simulink model "project_6"  (R2019a)
settings: Solver=VariableStepAuto  StartTime=0.0  StopTime=10.0  RelTol=1e-3
values from neighbouring files (symbols this model uses):
  Kd = 50    [project_7_run.m]    (also in project_8_run.m = 200)
  Ki = 300    [project_7_run.m]    (also in project_8_run.m = 200; project_9.m = 40)
  Kp = 350    [project_7_run.m]    (also in project_8_run.m = 300; project_9.m = 800)
settings Model: Creator=Nikita  LastModifiedBy=Nikita

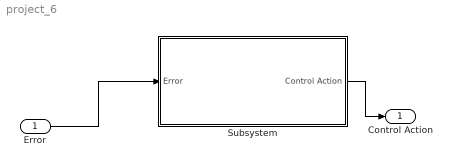
== system project_6 ==
  Error : Inport
  Subsystem : Subsystem
  Control Action : Outport
  wires:
  Error/1 -> Subsystem/1(Error)
  Subsystem/1(Control Action) -> Control Action/1

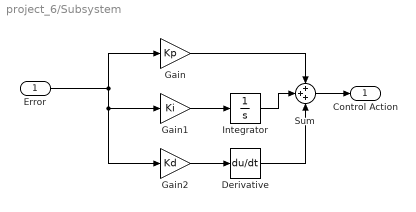
== system project_6/Subsystem ==
  Error : Inport
  Derivative : Derivative
  Gain : Gain  Gain=Kp
  Gain1 : Gain  Gain=Ki
  Gain2 : Gain  Gain=Kd
  Integrator : Integrator
  Sum : Sum  Inputs=+++
  Control Action : Outport
  wires:
  Gain2/1 -> Derivative/1
  Error/1 -> Gain2/1, Gain1/1, Gain/1
  Gain/1 -> Sum/1
  Derivative/1 -> Sum/3
  Gain1/1 -> Integrator/1
  Integrator/1 -> Sum/2
  Sum/1 -> Control Action/1
